simulink model "tongbukongzhi"  (R2022b)
settings: Solver=VariableStepAuto  StartTime=0.0  StopTime=10.0  RelTol=1e-3
values from neighbouring files (symbols this model uses):
  A = [-18/7 9 0;1 -1 1;0 -14.28 0]    [caishi.m]
  C = [1 0 0]    [caishi.m]
  H = [27/7;0;0]    [caishi.m]
settings Model: Creator=acer  LastModifiedBy=acer

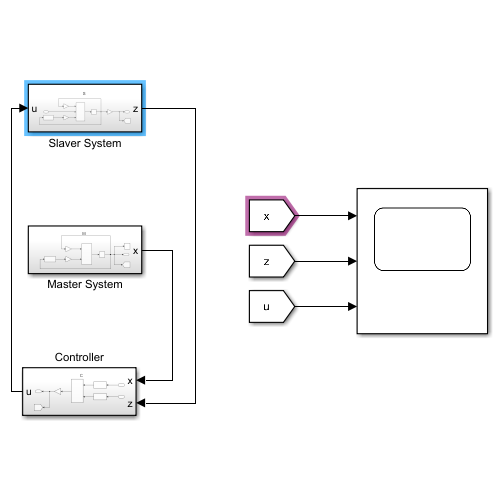
[thumbnail: Simulink's stored preview of the top-level diagram]
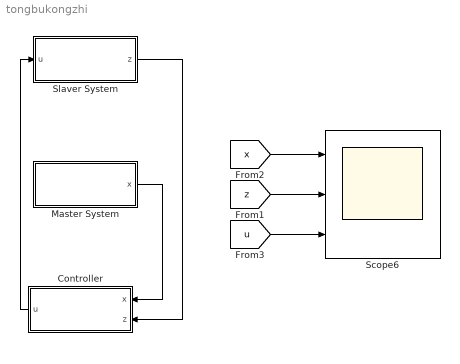
== system tongbukongzhi ==
  Controller : Subsystem
  Master System : Subsystem
  Scope6 : Scope  NumInputPorts=3
  Slaver System : Subsystem
  wires:
  [x] -> Scope6/1
  [z] -> Scope6/2
  Master System/1(x) -> Controller/1(x)
  [u] -> Scope6/3
  Controller/1(u) -> Slaver System/1(u)
  Slaver System/1(z) -> Controller/2(z)

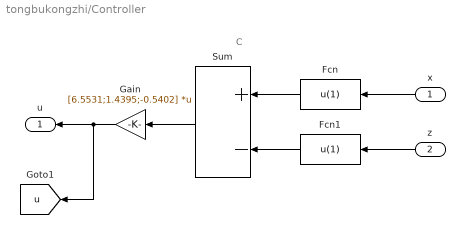
== system tongbukongzhi/Controller ==
  note: C
  x : Inport
  z : Inport  Port=2
  Fcn : Fcn  Expr=u(1)
  Fcn1 : Fcn  Expr=u(1)
  Gain : Gain  Gain=[6.5531;1.4395;-0.5402]  Multiplication=Matrix(K*u)
  Sum : Sum  Inputs=+-
  u : Outport
  tag scope: u=global
  wires:
  z/1 -> Fcn1/1
  x/1 -> Fcn/1
  Fcn/1 -> Sum/1
  Fcn1/1 -> Sum/2
  Sum/1 -> Gain/1
  Gain/1 -> [u], u/1

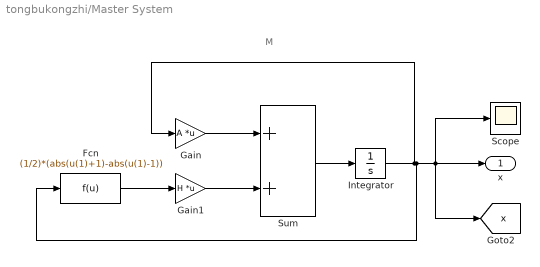
== system tongbukongzhi/Master System ==
  note: M
  Fcn : Fcn  Expr=(1/2)*(abs(u(1)+1)-abs(u(1)-1))
  Gain : Gain  Gain=A  Multiplication=Matrix(K*u)
  Gain1 : Gain  Gain=H  Multiplication=Matrix(K*u)
  Integrator : Integrator  InitialCondition=[-0.1;0.1;0.2]
  Scope : Scope
  Sum : Sum
  x : Outport
  tag scope: x=global
  wires:
  Gain/1 -> Sum/1
  Gain1/1 -> Sum/2
  Sum/1 -> Integrator/1
  Fcn/1 -> Gain1/1
  Integrator/1 -> x/1, Scope/1, [x], Fcn/1, Gain/1

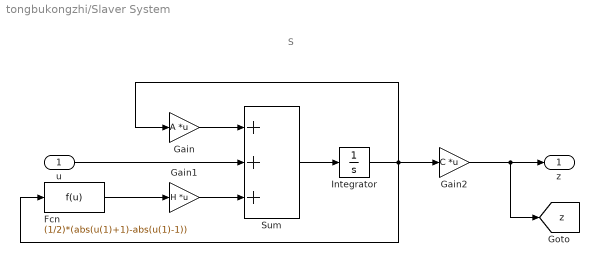
== system tongbukongzhi/Slaver System ==
  note: S
  u : Inport
  Fcn : Fcn  Expr=(1/2)*(abs(u(1)+1)-abs(u(1)-1))
  Gain : Gain  Gain=A  Multiplication=Matrix(K*u)
  Gain1 : Gain  Gain=H  Multiplication=Matrix(K*u)
  Gain2 : Gain  Gain=C  Multiplication=Matrix(K*u)
  Integrator : Integrator  InitialCondition=[0.2;0.3;0.7]
  Sum : Sum  Inputs=+++
  z : Outport
  tag scope: z=global
  wires:
  Gain/1 -> Sum/1
  Integrator/1 -> Fcn/1, Gain2/1, Gain/1
  Sum/1 -> Integrator/1
  Fcn/1 -> Gain1/1
  Gain1/1 -> Sum/3
  u/1 -> Sum/2
  Gain2/1 -> [z], z/1
